simulink model "WippleModel"  (R2018a)
settings: Solver=VariableStepAuto  StartTime=0.0  StopTime=7  MaxStep=0.01  RelTol=1e-3
undefined symbols (not defined in the file): C1, g, K0, K2, M
libraries: simulink_extras x2, simulink x1
settings Model: Creator=ProjectHT2018-2  LastModifiedBy=gct14001
settings DebuggingCC: LibraryContextMissingDiagnostic=warning
settings SFSimCC: SimUseLocalCustomCode=on
settings RTWCC: RTWUseLocalCustomCode=on

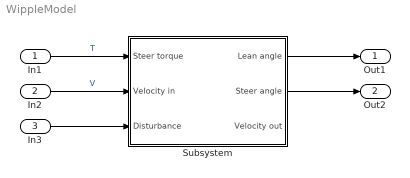
== system WippleModel ==
  In1 : Inport
  In2 : Inport  Port=2
  In3 : Inport  Port=3
  Subsystem : Subsystem
  Out1 : Outport
  Out2 : Outport  Port=2
  wires:
  In1/1 -> Subsystem/1(Steer torque)  "T"
  In2/1 -> Subsystem/2(Velocity in)  "V"
  In3/1 -> Subsystem/3(Disturbance)
  Subsystem/1("Lean angle ") -> Out1/1
  Subsystem/2(Steer angle) -> Out2/1

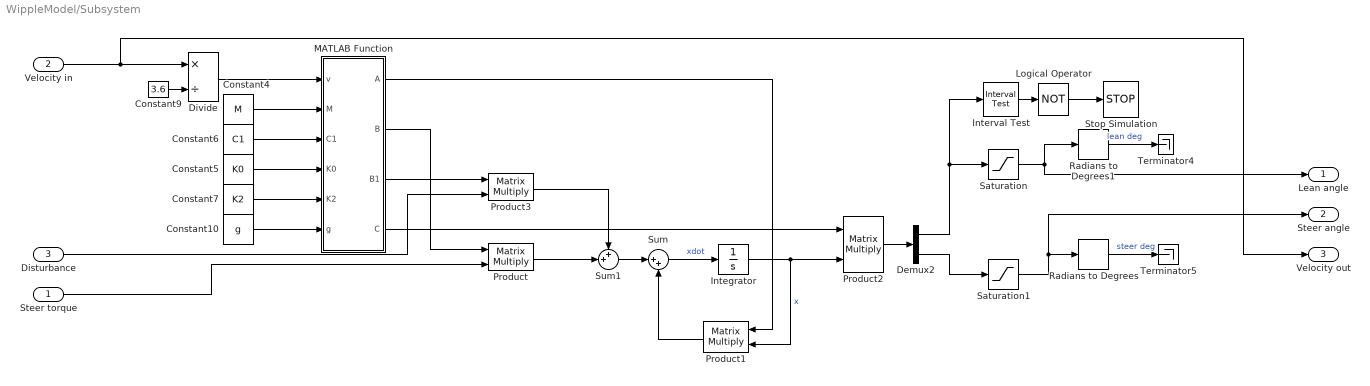
== system WippleModel/Subsystem ==
  Steer torque : Inport
  Velocity in : Inport  Port=2
  Disturbance : Inport  Port=3
  Constant10 : Constant  Value=g
  Constant4 : Constant  Value=M
  Constant5 : Constant  Value=K0
  Constant6 : Constant  Value=C1
  Constant7 : Constant  Value=K2
  Constant9 : Constant  Value=3.6
  Demux2 : Demux  Outputs=2
  Divide : Product  Inputs=*/
  Integrator : Integrator
  Interval Test : simulink/Logic and Bit Operations/Interval Test  IntervalClosedRight=on  uplimit=pi/4  IntervalClosedLeft=on  lowlimit=-pi/4  OutDataTypeStr=boolean
  Logical Operator : Logic  Operator=NOT  AllPortsSameDT=off  OutDataTypeStr=boolean
  MATLAB Function : MATLAB Function  TreatAsAtomicUnit=on
  Product{,1..3} (4 alike) : Product  Multiplication=Matrix(*)
  Radians to Degrees : simulink_extras/Transformations/Radians to Degrees
  Radians to Degrees1 : simulink_extras/Transformations/Radians to Degrees
  Saturation : Saturate  UpperLimit=pi/2  LowerLimit=-pi/2
  Saturation1 : Saturate  UpperLimit=pi/2  LowerLimit=-pi/2
  Stop Simulation : Stop
  Sum : Sum  Inputs=|++
  Sum1 : Sum  Inputs=++|
  Terminator4 : Terminator
  Terminator5 : Terminator
  "Lean angle " : Outport
  Steer angle : Outport  Port=2
  Velocity out : Outport  Port=3
  wires:
  Saturation/1 -> "Lean angle "/1, Radians to Degrees1/1
  Saturation1/1 -> Steer angle/1, Radians to Degrees/1
  Velocity in/1 -> Velocity out/1, Divide/1
  Demux2/1 -> Interval Test/1, Saturation/1
  Product/1 -> Sum1/2
  Product1/1 -> Sum/2
  Constant7/1 -> MATLAB Function/5(K2)
  MATLAB Function/2(B) -> Product/1
  Demux2/2 -> Saturation1/1
  Constant4/1 -> MATLAB Function/2(M)
  Radians to Degrees1/1 -> Terminator4/1  "lean deg"
  Sum/1 -> Integrator/1  "xdot"
  Constant5/1 -> MATLAB Function/4(K0)
  Sum1/1 -> Sum/1
  Constant6/1 -> MATLAB Function/3(C1)
  Disturbance/1 -> Product3/2
  Interval Test/1 -> Logical Operator/1
  Product2/1 -> Demux2/1
  Constant9/1 -> Divide/2
  Integrator/1 -> Product1/2, Product2/2  "x"
  Product3/1 -> Sum1/1
  MATLAB Function/3(B1) -> Product3/1
  Logical Operator/1 -> Stop Simulation/1
  MATLAB Function/1(A) -> Product1/1
  MATLAB Function/4(C) -> Product2/1
  Divide/1 -> MATLAB Function/1(v)
  Steer torque/1 -> Product/2
  Radians to Degrees/1 -> Terminator5/1  "steer deg"
  Constant10/1 -> MATLAB Function/6(g)

== matlab function WippleModel/Subsystem/MATLAB Function ==
  data: v input; A output; B output; B1 output; C output; M input; C1 input; K0 input; K2 input; g input
function [A,B,B1,C] = fcn(v, M, C1, K0, K2, g)

 %A matrix
 A1=[0 0; 0 0];
 A2=[1 0; 0 1];
 A3=-inv(M)*(g*K0+v^2*K2);
 A4=-inv(M)*v*C1;
 A=[A1, A2; A3, A4];
 
 %B matrix
 B=[[0; 0]; inv(M)*[0;1]]; 
 
 %B1 matrix
 B1=[[0; 0]; inv(M)*[1;0]]; 
  
 %C matrix
 C=[1 0 0 0; 0 1 0 0];
 
 %D matrix
 D=[0; 0];
